simulink model "can8auto"  (R2018a)
settings: Solver=VariableStepAuto  StartTime=0.0  StopTime=5000  RelTol=1e-3
libraries: commcrc2 x20, simulink x20, simulink_extras x5, dspswit3 x5
(part 6 of 7)

== system can8auto/PDO NODO CAN /CAN NODE/NMT Frame generator/11-bit Adder/11-bit Adder/Full Adder5 ==
  A : Inport
  B : Inport  Port=2
  Cin : Inport  Port=3
  AND : Logic  IconShape=distinctive  AllPortsSameDT=off  OutDataTypeStr=boolean
  AND1 : Logic  IconShape=distinctive  AllPortsSameDT=off  OutDataTypeStr=boolean
  OR : Logic  Operator=OR  IconShape=distinctive  AllPortsSameDT=off  OutDataTypeStr=boolean
  XOR1 : Logic  Operator=XOR  IconShape=distinctive  AllPortsSameDT=off  OutDataTypeStr=boolean
  XOR2 : Logic  Operator=XOR  IconShape=distinctive  AllPortsSameDT=off  OutDataTypeStr=boolean
  S : Outport
  Cout : Outport  Port=2
  wires:
  AND/1 -> OR/1
  XOR2/1 -> S/1
  B/1 -> XOR1/2, AND1/2
  A/1 -> XOR1/1, AND1/1
  AND1/1 -> OR/2
  XOR1/1 -> XOR2/1, AND/2
  Cin/1 -> AND/1, XOR2/2
  OR/1 -> Cout/1

== system can8auto/PDO NODO CAN /CAN NODE/NMT Frame generator/11-bit Adder/11-bit Adder/Full Adder6 ==
  A : Inport
  B : Inport  Port=2
  Cin : Inport  Port=3
  AND : Logic  IconShape=distinctive  AllPortsSameDT=off  OutDataTypeStr=boolean
  AND1 : Logic  IconShape=distinctive  AllPortsSameDT=off  OutDataTypeStr=boolean
  OR : Logic  Operator=OR  IconShape=distinctive  AllPortsSameDT=off  OutDataTypeStr=boolean
  XOR1 : Logic  Operator=XOR  IconShape=distinctive  AllPortsSameDT=off  OutDataTypeStr=boolean
  XOR2 : Logic  Operator=XOR  IconShape=distinctive  AllPortsSameDT=off  OutDataTypeStr=boolean
  S : Outport
  Cout : Outport  Port=2
  wires:
  AND/1 -> OR/1
  XOR2/1 -> S/1
  B/1 -> XOR1/2, AND1/2
  A/1 -> XOR1/1, AND1/1
  AND1/1 -> OR/2
  XOR1/1 -> XOR2/1, AND/2
  Cin/1 -> AND/1, XOR2/2
  OR/1 -> Cout/1

== system can8auto/PDO NODO CAN /CAN NODE/NMT Frame generator/11-bit Adder/11-bit Adder/Full Adder7 ==
  A : Inport
  B : Inport  Port=2
  Cin : Inport  Port=3
  AND : Logic  IconShape=distinctive  AllPortsSameDT=off  OutDataTypeStr=boolean
  AND1 : Logic  IconShape=distinctive  AllPortsSameDT=off  OutDataTypeStr=boolean
  OR : Logic  Operator=OR  IconShape=distinctive  AllPortsSameDT=off  OutDataTypeStr=boolean
  XOR1 : Logic  Operator=XOR  IconShape=distinctive  AllPortsSameDT=off  OutDataTypeStr=boolean
  XOR2 : Logic  Operator=XOR  IconShape=distinctive  AllPortsSameDT=off  OutDataTypeStr=boolean
  S : Outport
  Cout : Outport  Port=2
  wires:
  AND/1 -> OR/1
  XOR2/1 -> S/1
  B/1 -> XOR1/2, AND1/2
  A/1 -> XOR1/1, AND1/1
  AND1/1 -> OR/2
  XOR1/1 -> XOR2/1, AND/2
  Cin/1 -> AND/1, XOR2/2
  OR/1 -> Cout/1

== system can8auto/PDO NODO CAN /CAN NODE/NMT Frame generator/11-bit Adder/11-bit Adder/Full Adder8 ==
  A : Inport
  B : Inport  Port=2
  Cin : Inport  Port=3
  AND : Logic  IconShape=distinctive  AllPortsSameDT=off  OutDataTypeStr=boolean
  AND1 : Logic  IconShape=distinctive  AllPortsSameDT=off  OutDataTypeStr=boolean
  OR : Logic  Operator=OR  IconShape=distinctive  AllPortsSameDT=off  OutDataTypeStr=boolean
  XOR1 : Logic  Operator=XOR  IconShape=distinctive  AllPortsSameDT=off  OutDataTypeStr=boolean
  XOR2 : Logic  Operator=XOR  IconShape=distinctive  AllPortsSameDT=off  OutDataTypeStr=boolean
  S : Outport
  Cout : Outport  Port=2
  wires:
  AND/1 -> OR/1
  XOR2/1 -> S/1
  B/1 -> XOR1/2, AND1/2
  A/1 -> XOR1/1, AND1/1
  AND1/1 -> OR/2
  XOR1/1 -> XOR2/1, AND/2
  Cin/1 -> AND/1, XOR2/2
  OR/1 -> Cout/1

== system can8auto/PDO NODO CAN /CAN NODE/NMT Frame generator/11-bit Adder/11-bit Adder/Full Adder9 ==
  A : Inport
  B : Inport  Port=2
  Cin : Inport  Port=3
  AND : Logic  IconShape=distinctive  AllPortsSameDT=off  OutDataTypeStr=boolean
  AND1 : Logic  IconShape=distinctive  AllPortsSameDT=off  OutDataTypeStr=boolean
  OR : Logic  Operator=OR  IconShape=distinctive  AllPortsSameDT=off  OutDataTypeStr=boolean
  XOR1 : Logic  Operator=XOR  IconShape=distinctive  AllPortsSameDT=off  OutDataTypeStr=boolean
  XOR2 : Logic  Operator=XOR  IconShape=distinctive  AllPortsSameDT=off  OutDataTypeStr=boolean
  S : Outport
  Cout : Outport  Port=2
  wires:
  AND/1 -> OR/1
  XOR2/1 -> S/1
  B/1 -> XOR1/2, AND1/2
  A/1 -> XOR1/1, AND1/1
  AND1/1 -> OR/2
  XOR1/1 -> XOR2/1, AND/2
  Cin/1 -> AND/1, XOR2/2
  OR/1 -> Cout/1

== system can8auto/PDO NODO CAN /CAN NODE/NMT Frame generator/11-bit Adder/11-bit Adder/Half Adder ==
  A : Inport
  B : Inport  Port=2
  AND : Logic  IconShape=distinctive  AllPortsSameDT=off  OutDataTypeStr=boolean
  XOR1 : Logic  Operator=XOR  IconShape=distinctive  AllPortsSameDT=off  OutDataTypeStr=boolean
  S : Outport
  C : Outport  Port=2
  wires:
  A/1 -> XOR1/1, AND/1
  B/1 -> XOR1/2, AND/2
  AND/1 -> C/1
  XOR1/1 -> S/1

== system can8auto/SDO NODO CAN/CAN NODE/Bootup Frame generator/11-bit Adder/8-bit Adder/Full Adder ==
  A : Inport
  B : Inport  Port=2
  Cin : Inport  Port=3
  AND : Logic  IconShape=distinctive  AllPortsSameDT=off  OutDataTypeStr=boolean
  AND1 : Logic  IconShape=distinctive  AllPortsSameDT=off  OutDataTypeStr=boolean
  OR : Logic  Operator=OR  IconShape=distinctive  AllPortsSameDT=off  OutDataTypeStr=boolean
  XOR1 : Logic  Operator=XOR  IconShape=distinctive  AllPortsSameDT=off  OutDataTypeStr=boolean
  XOR2 : Logic  Operator=XOR  IconShape=distinctive  AllPortsSameDT=off  OutDataTypeStr=boolean
  S : Outport
  Cout : Outport  Port=2
  wires:
  AND/1 -> OR/1
  XOR2/1 -> S/1
  B/1 -> XOR1/2, AND1/2
  A/1 -> XOR1/1, AND1/1
  AND1/1 -> OR/2
  XOR1/1 -> XOR2/1, AND/2
  Cin/1 -> AND/1, XOR2/2
  OR/1 -> Cout/1

== system can8auto/SDO NODO CAN/CAN NODE/Bootup Frame generator/11-bit Adder/8-bit Adder/Full Adder1 ==
  A : Inport
  B : Inport  Port=2
  Cin : Inport  Port=3
  AND : Logic  IconShape=distinctive  AllPortsSameDT=off  OutDataTypeStr=boolean
  AND1 : Logic  IconShape=distinctive  AllPortsSameDT=off  OutDataTypeStr=boolean
  OR : Logic  Operator=OR  IconShape=distinctive  AllPortsSameDT=off  OutDataTypeStr=boolean
  XOR1 : Logic  Operator=XOR  IconShape=distinctive  AllPortsSameDT=off  OutDataTypeStr=boolean
  XOR2 : Logic  Operator=XOR  IconShape=distinctive  AllPortsSameDT=off  OutDataTypeStr=boolean
  S : Outport
  Cout : Outport  Port=2
  wires:
  AND/1 -> OR/1
  XOR2/1 -> S/1
  B/1 -> XOR1/2, AND1/2
  A/1 -> XOR1/1, AND1/1
  AND1/1 -> OR/2
  XOR1/1 -> XOR2/1, AND/2
  Cin/1 -> AND/1, XOR2/2
  OR/1 -> Cout/1

== system can8auto/SDO NODO CAN/CAN NODE/Bootup Frame generator/11-bit Adder/8-bit Adder/Full Adder2 ==
  A : Inport
  B : Inport  Port=2
  Cin : Inport  Port=3
  AND : Logic  IconShape=distinctive  AllPortsSameDT=off  OutDataTypeStr=boolean
  AND1 : Logic  IconShape=distinctive  AllPortsSameDT=off  OutDataTypeStr=boolean
  OR : Logic  Operator=OR  IconShape=distinctive  AllPortsSameDT=off  OutDataTypeStr=boolean
  XOR1 : Logic  Operator=XOR  IconShape=distinctive  AllPortsSameDT=off  OutDataTypeStr=boolean
  XOR2 : Logic  Operator=XOR  IconShape=distinctive  AllPortsSameDT=off  OutDataTypeStr=boolean
  S : Outport
  Cout : Outport  Port=2
  wires:
  AND/1 -> OR/1
  XOR2/1 -> S/1
  B/1 -> XOR1/2, AND1/2
  A/1 -> XOR1/1, AND1/1
  AND1/1 -> OR/2
  XOR1/1 -> XOR2/1, AND/2
  Cin/1 -> AND/1, XOR2/2
  OR/1 -> Cout/1

== system can8auto/SDO NODO CAN/CAN NODE/Bootup Frame generator/11-bit Adder/8-bit Adder/Full Adder3 ==
  A : Inport
  B : Inport  Port=2
  Cin : Inport  Port=3
  AND : Logic  IconShape=distinctive  AllPortsSameDT=off  OutDataTypeStr=boolean
  AND1 : Logic  IconShape=distinctive  AllPortsSameDT=off  OutDataTypeStr=boolean
  OR : Logic  Operator=OR  IconShape=distinctive  AllPortsSameDT=off  OutDataTypeStr=boolean
  XOR1 : Logic  Operator=XOR  IconShape=distinctive  AllPortsSameDT=off  OutDataTypeStr=boolean
  XOR2 : Logic  Operator=XOR  IconShape=distinctive  AllPortsSameDT=off  OutDataTypeStr=boolean
  S : Outport
  Cout : Outport  Port=2
  wires:
  AND/1 -> OR/1
  XOR2/1 -> S/1
  B/1 -> XOR1/2, AND1/2
  A/1 -> XOR1/1, AND1/1
  AND1/1 -> OR/2
  XOR1/1 -> XOR2/1, AND/2
  Cin/1 -> AND/1, XOR2/2
  OR/1 -> Cout/1

== system can8auto/SDO NODO CAN/CAN NODE/Bootup Frame generator/11-bit Adder/8-bit Adder/Full Adder4 ==
  A : Inport
  B : Inport  Port=2
  Cin : Inport  Port=3
  AND : Logic  IconShape=distinctive  AllPortsSameDT=off  OutDataTypeStr=boolean
  AND1 : Logic  IconShape=distinctive  AllPortsSameDT=off  OutDataTypeStr=boolean
  OR : Logic  Operator=OR  IconShape=distinctive  AllPortsSameDT=off  OutDataTypeStr=boolean
  XOR1 : Logic  Operator=XOR  IconShape=distinctive  AllPortsSameDT=off  OutDataTypeStr=boolean
  XOR2 : Logic  Operator=XOR  IconShape=distinctive  AllPortsSameDT=off  OutDataTypeStr=boolean
  S : Outport
  Cout : Outport  Port=2
  wires:
  AND/1 -> OR/1
  XOR2/1 -> S/1
  B/1 -> XOR1/2, AND1/2
  A/1 -> XOR1/1, AND1/1
  AND1/1 -> OR/2
  XOR1/1 -> XOR2/1, AND/2
  Cin/1 -> AND/1, XOR2/2
  OR/1 -> Cout/1

== system can8auto/SDO NODO CAN/CAN NODE/Bootup Frame generator/11-bit Adder/8-bit Adder/Full Adder5 ==
  A : Inport
  B : Inport  Port=2
  Cin : Inport  Port=3
  AND : Logic  IconShape=distinctive  AllPortsSameDT=off  OutDataTypeStr=boolean
  AND1 : Logic  IconShape=distinctive  AllPortsSameDT=off  OutDataTypeStr=boolean
  OR : Logic  Operator=OR  IconShape=distinctive  AllPortsSameDT=off  OutDataTypeStr=boolean
  XOR1 : Logic  Operator=XOR  IconShape=distinctive  AllPortsSameDT=off  OutDataTypeStr=boolean
  XOR2 : Logic  Operator=XOR  IconShape=distinctive  AllPortsSameDT=off  OutDataTypeStr=boolean
  S : Outport
  Cout : Outport  Port=2
  wires:
  AND/1 -> OR/1
  XOR2/1 -> S/1
  B/1 -> XOR1/2, AND1/2
  A/1 -> XOR1/1, AND1/1
  AND1/1 -> OR/2
  XOR1/1 -> XOR2/1, AND/2
  Cin/1 -> AND/1, XOR2/2
  OR/1 -> Cout/1

== system can8auto/SDO NODO CAN/CAN NODE/Bootup Frame generator/11-bit Adder/8-bit Adder/Full Adder6 ==
  A : Inport
  B : Inport  Port=2
  Cin : Inport  Port=3
  AND : Logic  IconShape=distinctive  AllPortsSameDT=off  OutDataTypeStr=boolean
  AND1 : Logic  IconShape=distinctive  AllPortsSameDT=off  OutDataTypeStr=boolean
  OR : Logic  Operator=OR  IconShape=distinctive  AllPortsSameDT=off  OutDataTypeStr=boolean
  XOR1 : Logic  Operator=XOR  IconShape=distinctive  AllPortsSameDT=off  OutDataTypeStr=boolean
  XOR2 : Logic  Operator=XOR  IconShape=distinctive  AllPortsSameDT=off  OutDataTypeStr=boolean
  S : Outport
  Cout : Outport  Port=2
  wires:
  AND/1 -> OR/1
  XOR2/1 -> S/1
  B/1 -> XOR1/2, AND1/2
  A/1 -> XOR1/1, AND1/1
  AND1/1 -> OR/2
  XOR1/1 -> XOR2/1, AND/2
  Cin/1 -> AND/1, XOR2/2
  OR/1 -> Cout/1

== system can8auto/SDO NODO CAN/CAN NODE/Bootup Frame generator/11-bit Adder/8-bit Adder/Full Adder7 ==
  A : Inport
  B : Inport  Port=2
  Cin : Inport  Port=3
  AND : Logic  IconShape=distinctive  AllPortsSameDT=off  OutDataTypeStr=boolean
  AND1 : Logic  IconShape=distinctive  AllPortsSameDT=off  OutDataTypeStr=boolean
  OR : Logic  Operator=OR  IconShape=distinctive  AllPortsSameDT=off  OutDataTypeStr=boolean
  XOR1 : Logic  Operator=XOR  IconShape=distinctive  AllPortsSameDT=off  OutDataTypeStr=boolean
  XOR2 : Logic  Operator=XOR  IconShape=distinctive  AllPortsSameDT=off  OutDataTypeStr=boolean
  S : Outport
  Cout : Outport  Port=2
  wires:
  AND/1 -> OR/1
  XOR2/1 -> S/1
  B/1 -> XOR1/2, AND1/2
  A/1 -> XOR1/1, AND1/1
  AND1/1 -> OR/2
  XOR1/1 -> XOR2/1, AND/2
  Cin/1 -> AND/1, XOR2/2
  OR/1 -> Cout/1

== system can8auto/SDO NODO CAN/CAN NODE/Bootup Frame generator/11-bit Adder/8-bit Adder/Full Adder8 ==
  A : Inport
  B : Inport  Port=2
  Cin : Inport  Port=3
  AND : Logic  IconShape=distinctive  AllPortsSameDT=off  OutDataTypeStr=boolean
  AND1 : Logic  IconShape=distinctive  AllPortsSameDT=off  OutDataTypeStr=boolean
  OR : Logic  Operator=OR  IconShape=distinctive  AllPortsSameDT=off  OutDataTypeStr=boolean
  XOR1 : Logic  Operator=XOR  IconShape=distinctive  AllPortsSameDT=off  OutDataTypeStr=boolean
  XOR2 : Logic  Operator=XOR  IconShape=distinctive  AllPortsSameDT=off  OutDataTypeStr=boolean
  S : Outport
  Cout : Outport  Port=2
  wires:
  AND/1 -> OR/1
  XOR2/1 -> S/1
  B/1 -> XOR1/2, AND1/2
  A/1 -> XOR1/1, AND1/1
  AND1/1 -> OR/2
  XOR1/1 -> XOR2/1, AND/2
  Cin/1 -> AND/1, XOR2/2
  OR/1 -> Cout/1

== system can8auto/SDO NODO CAN/CAN NODE/Bootup Frame generator/11-bit Adder/8-bit Adder/Full Adder9 ==
  A : Inport
  B : Inport  Port=2
  Cin : Inport  Port=3
  AND : Logic  IconShape=distinctive  AllPortsSameDT=off  OutDataTypeStr=boolean
  AND1 : Logic  IconShape=distinctive  AllPortsSameDT=off  OutDataTypeStr=boolean
  OR : Logic  Operator=OR  IconShape=distinctive  AllPortsSameDT=off  OutDataTypeStr=boolean
  XOR1 : Logic  Operator=XOR  IconShape=distinctive  AllPortsSameDT=off  OutDataTypeStr=boolean
  XOR2 : Logic  Operator=XOR  IconShape=distinctive  AllPortsSameDT=off  OutDataTypeStr=boolean
  S : Outport
  Cout : Outport  Port=2
  wires:
  AND/1 -> OR/1
  XOR2/1 -> S/1
  B/1 -> XOR1/2, AND1/2
  A/1 -> XOR1/1, AND1/1
  AND1/1 -> OR/2
  XOR1/1 -> XOR2/1, AND/2
  Cin/1 -> AND/1, XOR2/2
  OR/1 -> Cout/1

== system can8auto/SDO NODO CAN/CAN NODE/Bootup Frame generator/11-bit Adder/8-bit Adder/Half Adder ==
  A : Inport
  B : Inport  Port=2
  AND : Logic  IconShape=distinctive  AllPortsSameDT=off  OutDataTypeStr=boolean
  XOR1 : Logic  Operator=XOR  IconShape=distinctive  AllPortsSameDT=off  OutDataTypeStr=boolean
  S : Outport
  C : Outport  Port=2
  wires:
  A/1 -> XOR1/1, AND/1
  B/1 -> XOR1/2, AND/2
  AND/1 -> C/1
  XOR1/1 -> S/1

== system can8auto/SDO NODO CAN/CAN NODE/NMT Frame generator/11-bit Adder/11-bit Adder/Full Adder ==
  A : Inport
  B : Inport  Port=2
  Cin : Inport  Port=3
  AND : Logic  IconShape=distinctive  AllPortsSameDT=off  OutDataTypeStr=boolean
  AND1 : Logic  IconShape=distinctive  AllPortsSameDT=off  OutDataTypeStr=boolean
  OR : Logic  Operator=OR  IconShape=distinctive  AllPortsSameDT=off  OutDataTypeStr=boolean
  XOR1 : Logic  Operator=XOR  IconShape=distinctive  AllPortsSameDT=off  OutDataTypeStr=boolean
  XOR2 : Logic  Operator=XOR  IconShape=distinctive  AllPortsSameDT=off  OutDataTypeStr=boolean
  S : Outport
  Cout : Outport  Port=2
  wires:
  AND/1 -> OR/1
  XOR2/1 -> S/1
  B/1 -> XOR1/2, AND1/2
  A/1 -> XOR1/1, AND1/1
  AND1/1 -> OR/2
  XOR1/1 -> XOR2/1, AND/2
  Cin/1 -> AND/1, XOR2/2
  OR/1 -> Cout/1

== system can8auto/SDO NODO CAN/CAN NODE/NMT Frame generator/11-bit Adder/11-bit Adder/Full Adder1 ==
  A : Inport
  B : Inport  Port=2
  Cin : Inport  Port=3
  AND : Logic  IconShape=distinctive  AllPortsSameDT=off  OutDataTypeStr=boolean
  AND1 : Logic  IconShape=distinctive  AllPortsSameDT=off  OutDataTypeStr=boolean
  OR : Logic  Operator=OR  IconShape=distinctive  AllPortsSameDT=off  OutDataTypeStr=boolean
  XOR1 : Logic  Operator=XOR  IconShape=distinctive  AllPortsSameDT=off  OutDataTypeStr=boolean
  XOR2 : Logic  Operator=XOR  IconShape=distinctive  AllPortsSameDT=off  OutDataTypeStr=boolean
  S : Outport
  Cout : Outport  Port=2
  wires:
  AND/1 -> OR/1
  XOR2/1 -> S/1
  B/1 -> XOR1/2, AND1/2
  A/1 -> XOR1/1, AND1/1
  AND1/1 -> OR/2
  XOR1/1 -> XOR2/1, AND/2
  Cin/1 -> AND/1, XOR2/2
  OR/1 -> Cout/1

== system can8auto/SDO NODO CAN/CAN NODE/NMT Frame generator/11-bit Adder/11-bit Adder/Full Adder2 ==
  A : Inport
  B : Inport  Port=2
  Cin : Inport  Port=3
  AND : Logic  IconShape=distinctive  AllPortsSameDT=off  OutDataTypeStr=boolean
  AND1 : Logic  IconShape=distinctive  AllPortsSameDT=off  OutDataTypeStr=boolean
  OR : Logic  Operator=OR  IconShape=distinctive  AllPortsSameDT=off  OutDataTypeStr=boolean
  XOR1 : Logic  Operator=XOR  IconShape=distinctive  AllPortsSameDT=off  OutDataTypeStr=boolean
  XOR2 : Logic  Operator=XOR  IconShape=distinctive  AllPortsSameDT=off  OutDataTypeStr=boolean
  S : Outport
  Cout : Outport  Port=2
  wires:
  AND/1 -> OR/1
  XOR2/1 -> S/1
  B/1 -> XOR1/2, AND1/2
  A/1 -> XOR1/1, AND1/1
  AND1/1 -> OR/2
  XOR1/1 -> XOR2/1, AND/2
  Cin/1 -> AND/1, XOR2/2
  OR/1 -> Cout/1

== system can8auto/SDO NODO CAN/CAN NODE/NMT Frame generator/11-bit Adder/11-bit Adder/Full Adder3 ==
  A : Inport
  B : Inport  Port=2
  Cin : Inport  Port=3
  AND : Logic  IconShape=distinctive  AllPortsSameDT=off  OutDataTypeStr=boolean
  AND1 : Logic  IconShape=distinctive  AllPortsSameDT=off  OutDataTypeStr=boolean
  OR : Logic  Operator=OR  IconShape=distinctive  AllPortsSameDT=off  OutDataTypeStr=boolean
  XOR1 : Logic  Operator=XOR  IconShape=distinctive  AllPortsSameDT=off  OutDataTypeStr=boolean
  XOR2 : Logic  Operator=XOR  IconShape=distinctive  AllPortsSameDT=off  OutDataTypeStr=boolean
  S : Outport
  Cout : Outport  Port=2
  wires:
  AND/1 -> OR/1
  XOR2/1 -> S/1
  B/1 -> XOR1/2, AND1/2
  A/1 -> XOR1/1, AND1/1
  AND1/1 -> OR/2
  XOR1/1 -> XOR2/1, AND/2
  Cin/1 -> AND/1, XOR2/2
  OR/1 -> Cout/1

== system can8auto/SDO NODO CAN/CAN NODE/NMT Frame generator/11-bit Adder/11-bit Adder/Full Adder4 ==
  A : Inport
  B : Inport  Port=2
  Cin : Inport  Port=3
  AND : Logic  IconShape=distinctive  AllPortsSameDT=off  OutDataTypeStr=boolean
  AND1 : Logic  IconShape=distinctive  AllPortsSameDT=off  OutDataTypeStr=boolean
  OR : Logic  Operator=OR  IconShape=distinctive  AllPortsSameDT=off  OutDataTypeStr=boolean
  XOR1 : Logic  Operator=XOR  IconShape=distinctive  AllPortsSameDT=off  OutDataTypeStr=boolean
  XOR2 : Logic  Operator=XOR  IconShape=distinctive  AllPortsSameDT=off  OutDataTypeStr=boolean
  S : Outport
  Cout : Outport  Port=2
  wires:
  AND/1 -> OR/1
  XOR2/1 -> S/1
  B/1 -> XOR1/2, AND1/2
  A/1 -> XOR1/1, AND1/1
  AND1/1 -> OR/2
  XOR1/1 -> XOR2/1, AND/2
  Cin/1 -> AND/1, XOR2/2
  OR/1 -> Cout/1

== system can8auto/SDO NODO CAN/CAN NODE/NMT Frame generator/11-bit Adder/11-bit Adder/Full Adder5 ==
  A : Inport
  B : Inport  Port=2
  Cin : Inport  Port=3
  AND : Logic  IconShape=distinctive  AllPortsSameDT=off  OutDataTypeStr=boolean
  AND1 : Logic  IconShape=distinctive  AllPortsSameDT=off  OutDataTypeStr=boolean
  OR : Logic  Operator=OR  IconShape=distinctive  AllPortsSameDT=off  OutDataTypeStr=boolean
  XOR1 : Logic  Operator=XOR  IconShape=distinctive  AllPortsSameDT=off  OutDataTypeStr=boolean
  XOR2 : Logic  Operator=XOR  IconShape=distinctive  AllPortsSameDT=off  OutDataTypeStr=boolean
  S : Outport
  Cout : Outport  Port=2
  wires:
  AND/1 -> OR/1
  XOR2/1 -> S/1
  B/1 -> XOR1/2, AND1/2
  A/1 -> XOR1/1, AND1/1
  AND1/1 -> OR/2
  XOR1/1 -> XOR2/1, AND/2
  Cin/1 -> AND/1, XOR2/2
  OR/1 -> Cout/1

== system can8auto/SDO NODO CAN/CAN NODE/NMT Frame generator/11-bit Adder/11-bit Adder/Full Adder6 ==
  A : Inport
  B : Inport  Port=2
  Cin : Inport  Port=3
  AND : Logic  IconShape=distinctive  AllPortsSameDT=off  OutDataTypeStr=boolean
  AND1 : Logic  IconShape=distinctive  AllPortsSameDT=off  OutDataTypeStr=boolean
  OR : Logic  Operator=OR  IconShape=distinctive  AllPortsSameDT=off  OutDataTypeStr=boolean
  XOR1 : Logic  Operator=XOR  IconShape=distinctive  AllPortsSameDT=off  OutDataTypeStr=boolean
  XOR2 : Logic  Operator=XOR  IconShape=distinctive  AllPortsSameDT=off  OutDataTypeStr=boolean
  S : Outport
  Cout : Outport  Port=2
  wires:
  AND/1 -> OR/1
  XOR2/1 -> S/1
  B/1 -> XOR1/2, AND1/2
  A/1 -> XOR1/1, AND1/1
  AND1/1 -> OR/2
  XOR1/1 -> XOR2/1, AND/2
  Cin/1 -> AND/1, XOR2/2
  OR/1 -> Cout/1

== system can8auto/SDO NODO CAN/CAN NODE/NMT Frame generator/11-bit Adder/11-bit Adder/Full Adder7 ==
  A : Inport
  B : Inport  Port=2
  Cin : Inport  Port=3
  AND : Logic  IconShape=distinctive  AllPortsSameDT=off  OutDataTypeStr=boolean
  AND1 : Logic  IconShape=distinctive  AllPortsSameDT=off  OutDataTypeStr=boolean
  OR : Logic  Operator=OR  IconShape=distinctive  AllPortsSameDT=off  OutDataTypeStr=boolean
  XOR1 : Logic  Operator=XOR  IconShape=distinctive  AllPortsSameDT=off  OutDataTypeStr=boolean
  XOR2 : Logic  Operator=XOR  IconShape=distinctive  AllPortsSameDT=off  OutDataTypeStr=boolean
  S : Outport
  Cout : Outport  Port=2
  wires:
  AND/1 -> OR/1
  XOR2/1 -> S/1
  B/1 -> XOR1/2, AND1/2
  A/1 -> XOR1/1, AND1/1
  AND1/1 -> OR/2
  XOR1/1 -> XOR2/1, AND/2
  Cin/1 -> AND/1, XOR2/2
  OR/1 -> Cout/1

== system can8auto/SDO NODO CAN/CAN NODE/NMT Frame generator/11-bit Adder/11-bit Adder/Full Adder8 ==
  A : Inport
  B : Inport  Port=2
  Cin : Inport  Port=3
  AND : Logic  IconShape=distinctive  AllPortsSameDT=off  OutDataTypeStr=boolean
  AND1 : Logic  IconShape=distinctive  AllPortsSameDT=off  OutDataTypeStr=boolean
  OR : Logic  Operator=OR  IconShape=distinctive  AllPortsSameDT=off  OutDataTypeStr=boolean
  XOR1 : Logic  Operator=XOR  IconShape=distinctive  AllPortsSameDT=off  OutDataTypeStr=boolean
  XOR2 : Logic  Operator=XOR  IconShape=distinctive  AllPortsSameDT=off  OutDataTypeStr=boolean
  S : Outport
  Cout : Outport  Port=2
  wires:
  AND/1 -> OR/1
  XOR2/1 -> S/1
  B/1 -> XOR1/2, AND1/2
  A/1 -> XOR1/1, AND1/1
  AND1/1 -> OR/2
  XOR1/1 -> XOR2/1, AND/2
  Cin/1 -> AND/1, XOR2/2
  OR/1 -> Cout/1

== system can8auto/SDO NODO CAN/CAN NODE/NMT Frame generator/11-bit Adder/11-bit Adder/Full Adder9 ==
  A : Inport
  B : Inport  Port=2
  Cin : Inport  Port=3
  AND : Logic  IconShape=distinctive  AllPortsSameDT=off  OutDataTypeStr=boolean
  AND1 : Logic  IconShape=distinctive  AllPortsSameDT=off  OutDataTypeStr=boolean
  OR : Logic  Operator=OR  IconShape=distinctive  AllPortsSameDT=off  OutDataTypeStr=boolean
  XOR1 : Logic  Operator=XOR  IconShape=distinctive  AllPortsSameDT=off  OutDataTypeStr=boolean
  XOR2 : Logic  Operator=XOR  IconShape=distinctive  AllPortsSameDT=off  OutDataTypeStr=boolean
  S : Outport
  Cout : Outport  Port=2
  wires:
  AND/1 -> OR/1
  XOR2/1 -> S/1
  B/1 -> XOR1/2, AND1/2
  A/1 -> XOR1/1, AND1/1
  AND1/1 -> OR/2
  XOR1/1 -> XOR2/1, AND/2
  Cin/1 -> AND/1, XOR2/2
  OR/1 -> Cout/1

== system can8auto/SDO NODO CAN/CAN NODE/NMT Frame generator/11-bit Adder/11-bit Adder/Half Adder ==
  A : Inport
  B : Inport  Port=2
  AND : Logic  IconShape=distinctive  AllPortsSameDT=off  OutDataTypeStr=boolean
  XOR1 : Logic  Operator=XOR  IconShape=distinctive  AllPortsSameDT=off  OutDataTypeStr=boolean
  S : Outport
  C : Outport  Port=2
  wires:
  A/1 -> XOR1/1, AND/1
  B/1 -> XOR1/2, AND/2
  AND/1 -> C/1
  XOR1/1 -> S/1

== system can8auto/SYNC PRODUCER/CAN NODE/Bootup Frame generator/11-bit Adder/8-bit Adder/Full Adder ==
  A : Inport
  B : Inport  Port=2
  Cin : Inport  Port=3
  AND : Logic  IconShape=distinctive  AllPortsSameDT=off  OutDataTypeStr=boolean
  AND1 : Logic  IconShape=distinctive  AllPortsSameDT=off  OutDataTypeStr=boolean
  OR : Logic  Operator=OR  IconShape=distinctive  AllPortsSameDT=off  OutDataTypeStr=boolean
  XOR1 : Logic  Operator=XOR  IconShape=distinctive  AllPortsSameDT=off  OutDataTypeStr=boolean
  XOR2 : Logic  Operator=XOR  IconShape=distinctive  AllPortsSameDT=off  OutDataTypeStr=boolean
  S : Outport
  Cout : Outport  Port=2
  wires:
  AND/1 -> OR/1
  XOR2/1 -> S/1
  B/1 -> XOR1/2, AND1/2
  A/1 -> XOR1/1, AND1/1
  AND1/1 -> OR/2
  XOR1/1 -> XOR2/1, AND/2
  Cin/1 -> AND/1, XOR2/2
  OR/1 -> Cout/1

== system can8auto/SYNC PRODUCER/CAN NODE/Bootup Frame generator/11-bit Adder/8-bit Adder/Full Adder1 ==
  A : Inport
  B : Inport  Port=2
  Cin : Inport  Port=3
  AND : Logic  IconShape=distinctive  AllPortsSameDT=off  OutDataTypeStr=boolean
  AND1 : Logic  IconShape=distinctive  AllPortsSameDT=off  OutDataTypeStr=boolean
  OR : Logic  Operator=OR  IconShape=distinctive  AllPortsSameDT=off  OutDataTypeStr=boolean
  XOR1 : Logic  Operator=XOR  IconShape=distinctive  AllPortsSameDT=off  OutDataTypeStr=boolean
  XOR2 : Logic  Operator=XOR  IconShape=distinctive  AllPortsSameDT=off  OutDataTypeStr=boolean
  S : Outport
  Cout : Outport  Port=2
  wires:
  AND/1 -> OR/1
  XOR2/1 -> S/1
  B/1 -> XOR1/2, AND1/2
  A/1 -> XOR1/1, AND1/1
  AND1/1 -> OR/2
  XOR1/1 -> XOR2/1, AND/2
  Cin/1 -> AND/1, XOR2/2
  OR/1 -> Cout/1

== system can8auto/SYNC PRODUCER/CAN NODE/Bootup Frame generator/11-bit Adder/8-bit Adder/Full Adder2 ==
  A : Inport
  B : Inport  Port=2
  Cin : Inport  Port=3
  AND : Logic  IconShape=distinctive  AllPortsSameDT=off  OutDataTypeStr=boolean
  AND1 : Logic  IconShape=distinctive  AllPortsSameDT=off  OutDataTypeStr=boolean
  OR : Logic  Operator=OR  IconShape=distinctive  AllPortsSameDT=off  OutDataTypeStr=boolean
  XOR1 : Logic  Operator=XOR  IconShape=distinctive  AllPortsSameDT=off  OutDataTypeStr=boolean
  XOR2 : Logic  Operator=XOR  IconShape=distinctive  AllPortsSameDT=off  OutDataTypeStr=boolean
  S : Outport
  Cout : Outport  Port=2
  wires:
  AND/1 -> OR/1
  XOR2/1 -> S/1
  B/1 -> XOR1/2, AND1/2
  A/1 -> XOR1/1, AND1/1
  AND1/1 -> OR/2
  XOR1/1 -> XOR2/1, AND/2
  Cin/1 -> AND/1, XOR2/2
  OR/1 -> Cout/1

== system can8auto/SYNC PRODUCER/CAN NODE/Bootup Frame generator/11-bit Adder/8-bit Adder/Full Adder3 ==
  A : Inport
  B : Inport  Port=2
  Cin : Inport  Port=3
  AND : Logic  IconShape=distinctive  AllPortsSameDT=off  OutDataTypeStr=boolean
  AND1 : Logic  IconShape=distinctive  AllPortsSameDT=off  OutDataTypeStr=boolean
  OR : Logic  Operator=OR  IconShape=distinctive  AllPortsSameDT=off  OutDataTypeStr=boolean
  XOR1 : Logic  Operator=XOR  IconShape=distinctive  AllPortsSameDT=off  OutDataTypeStr=boolean
  XOR2 : Logic  Operator=XOR  IconShape=distinctive  AllPortsSameDT=off  OutDataTypeStr=boolean
  S : Outport
  Cout : Outport  Port=2
  wires:
  AND/1 -> OR/1
  XOR2/1 -> S/1
  B/1 -> XOR1/2, AND1/2
  A/1 -> XOR1/1, AND1/1
  AND1/1 -> OR/2
  XOR1/1 -> XOR2/1, AND/2
  Cin/1 -> AND/1, XOR2/2
  OR/1 -> Cout/1

== system can8auto/SYNC PRODUCER/CAN NODE/Bootup Frame generator/11-bit Adder/8-bit Adder/Full Adder4 ==
  A : Inport
  B : Inport  Port=2
  Cin : Inport  Port=3
  AND : Logic  IconShape=distinctive  AllPortsSameDT=off  OutDataTypeStr=boolean
  AND1 : Logic  IconShape=distinctive  AllPortsSameDT=off  OutDataTypeStr=boolean
  OR : Logic  Operator=OR  IconShape=distinctive  AllPortsSameDT=off  OutDataTypeStr=boolean
  XOR1 : Logic  Operator=XOR  IconShape=distinctive  AllPortsSameDT=off  OutDataTypeStr=boolean
  XOR2 : Logic  Operator=XOR  IconShape=distinctive  AllPortsSameDT=off  OutDataTypeStr=boolean
  S : Outport
  Cout : Outport  Port=2
  wires:
  AND/1 -> OR/1
  XOR2/1 -> S/1
  B/1 -> XOR1/2, AND1/2
  A/1 -> XOR1/1, AND1/1
  AND1/1 -> OR/2
  XOR1/1 -> XOR2/1, AND/2
  Cin/1 -> AND/1, XOR2/2
  OR/1 -> Cout/1

== system can8auto/SYNC PRODUCER/CAN NODE/Bootup Frame generator/11-bit Adder/8-bit Adder/Full Adder5 ==
  A : Inport
  B : Inport  Port=2
  Cin : Inport  Port=3
  AND : Logic  IconShape=distinctive  AllPortsSameDT=off  OutDataTypeStr=boolean
  AND1 : Logic  IconShape=distinctive  AllPortsSameDT=off  OutDataTypeStr=boolean
  OR : Logic  Operator=OR  IconShape=distinctive  AllPortsSameDT=off  OutDataTypeStr=boolean
  XOR1 : Logic  Operator=XOR  IconShape=distinctive  AllPortsSameDT=off  OutDataTypeStr=boolean
  XOR2 : Logic  Operator=XOR  IconShape=distinctive  AllPortsSameDT=off  OutDataTypeStr=boolean
  S : Outport
  Cout : Outport  Port=2
  wires:
  AND/1 -> OR/1
  XOR2/1 -> S/1
  B/1 -> XOR1/2, AND1/2
  A/1 -> XOR1/1, AND1/1
  AND1/1 -> OR/2
  XOR1/1 -> XOR2/1, AND/2
  Cin/1 -> AND/1, XOR2/2
  OR/1 -> Cout/1

== system can8auto/SYNC PRODUCER/CAN NODE/Bootup Frame generator/11-bit Adder/8-bit Adder/Full Adder6 ==
  A : Inport
  B : Inport  Port=2
  Cin : Inport  Port=3
  AND : Logic  IconShape=distinctive  AllPortsSameDT=off  OutDataTypeStr=boolean
  AND1 : Logic  IconShape=distinctive  AllPortsSameDT=off  OutDataTypeStr=boolean
  OR : Logic  Operator=OR  IconShape=distinctive  AllPortsSameDT=off  OutDataTypeStr=boolean
  XOR1 : Logic  Operator=XOR  IconShape=distinctive  AllPortsSameDT=off  OutDataTypeStr=boolean
  XOR2 : Logic  Operator=XOR  IconShape=distinctive  AllPortsSameDT=off  OutDataTypeStr=boolean
  S : Outport
  Cout : Outport  Port=2
  wires:
  AND/1 -> OR/1
  XOR2/1 -> S/1
  B/1 -> XOR1/2, AND1/2
  A/1 -> XOR1/1, AND1/1
  AND1/1 -> OR/2
  XOR1/1 -> XOR2/1, AND/2
  Cin/1 -> AND/1, XOR2/2
  OR/1 -> Cout/1

== system can8auto/SYNC PRODUCER/CAN NODE/Bootup Frame generator/11-bit Adder/8-bit Adder/Full Adder7 ==
  A : Inport
  B : Inport  Port=2
  Cin : Inport  Port=3
  AND : Logic  IconShape=distinctive  AllPortsSameDT=off  OutDataTypeStr=boolean
  AND1 : Logic  IconShape=distinctive  AllPortsSameDT=off  OutDataTypeStr=boolean
  OR : Logic  Operator=OR  IconShape=distinctive  AllPortsSameDT=off  OutDataTypeStr=boolean
  XOR1 : Logic  Operator=XOR  IconShape=distinctive  AllPortsSameDT=off  OutDataTypeStr=boolean
  XOR2 : Logic  Operator=XOR  IconShape=distinctive  AllPortsSameDT=off  OutDataTypeStr=boolean
  S : Outport
  Cout : Outport  Port=2
  wires:
  AND/1 -> OR/1
  XOR2/1 -> S/1
  B/1 -> XOR1/2, AND1/2
  A/1 -> XOR1/1, AND1/1
  AND1/1 -> OR/2
  XOR1/1 -> XOR2/1, AND/2
  Cin/1 -> AND/1, XOR2/2
  OR/1 -> Cout/1

== system can8auto/SYNC PRODUCER/CAN NODE/Bootup Frame generator/11-bit Adder/8-bit Adder/Full Adder8 ==
  A : Inport
  B : Inport  Port=2
  Cin : Inport  Port=3
  AND : Logic  IconShape=distinctive  AllPortsSameDT=off  OutDataTypeStr=boolean
  AND1 : Logic  IconShape=distinctive  AllPortsSameDT=off  OutDataTypeStr=boolean
  OR : Logic  Operator=OR  IconShape=distinctive  AllPortsSameDT=off  OutDataTypeStr=boolean
  XOR1 : Logic  Operator=XOR  IconShape=distinctive  AllPortsSameDT=off  OutDataTypeStr=boolean
  XOR2 : Logic  Operator=XOR  IconShape=distinctive  AllPortsSameDT=off  OutDataTypeStr=boolean
  S : Outport
  Cout : Outport  Port=2
  wires:
  AND/1 -> OR/1
  XOR2/1 -> S/1
  B/1 -> XOR1/2, AND1/2
  A/1 -> XOR1/1, AND1/1
  AND1/1 -> OR/2
  XOR1/1 -> XOR2/1, AND/2
  Cin/1 -> AND/1, XOR2/2
  OR/1 -> Cout/1

== system can8auto/SYNC PRODUCER/CAN NODE/Bootup Frame generator/11-bit Adder/8-bit Adder/Full Adder9 ==
  A : Inport
  B : Inport  Port=2
  Cin : Inport  Port=3
  AND : Logic  IconShape=distinctive  AllPortsSameDT=off  OutDataTypeStr=boolean
  AND1 : Logic  IconShape=distinctive  AllPortsSameDT=off  OutDataTypeStr=boolean
  OR : Logic  Operator=OR  IconShape=distinctive  AllPortsSameDT=off  OutDataTypeStr=boolean
  XOR1 : Logic  Operator=XOR  IconShape=distinctive  AllPortsSameDT=off  OutDataTypeStr=boolean
  XOR2 : Logic  Operator=XOR  IconShape=distinctive  AllPortsSameDT=off  OutDataTypeStr=boolean
  S : Outport
  Cout : Outport  Port=2
  wires:
  AND/1 -> OR/1
  XOR2/1 -> S/1
  B/1 -> XOR1/2, AND1/2
  A/1 -> XOR1/1, AND1/1
  AND1/1 -> OR/2
  XOR1/1 -> XOR2/1, AND/2
  Cin/1 -> AND/1, XOR2/2
  OR/1 -> Cout/1

== system can8auto/SYNC PRODUCER/CAN NODE/Bootup Frame generator/11-bit Adder/8-bit Adder/Half Adder ==
  A : Inport
  B : Inport  Port=2
  AND : Logic  IconShape=distinctive  AllPortsSameDT=off  OutDataTypeStr=boolean
  XOR1 : Logic  Operator=XOR  IconShape=distinctive  AllPortsSameDT=off  OutDataTypeStr=boolean
  S : Outport
  C : Outport  Port=2
  wires:
  A/1 -> XOR1/1, AND/1
  B/1 -> XOR1/2, AND/2
  AND/1 -> C/1
  XOR1/1 -> S/1

== system can8auto/SYNC PRODUCER/CAN NODE/NMT Frame generator/11-bit Adder/11-bit Adder/Full Adder ==
  A : Inport
  B : Inport  Port=2
  Cin : Inport  Port=3
  AND : Logic  IconShape=distinctive  AllPortsSameDT=off  OutDataTypeStr=boolean
  AND1 : Logic  IconShape=distinctive  AllPortsSameDT=off  OutDataTypeStr=boolean
  OR : Logic  Operator=OR  IconShape=distinctive  AllPortsSameDT=off  OutDataTypeStr=boolean
  XOR1 : Logic  Operator=XOR  IconShape=distinctive  AllPortsSameDT=off  OutDataTypeStr=boolean
  XOR2 : Logic  Operator=XOR  IconShape=distinctive  AllPortsSameDT=off  OutDataTypeStr=boolean
  S : Outport
  Cout : Outport  Port=2
  wires:
  AND/1 -> OR/1
  XOR2/1 -> S/1
  B/1 -> XOR1/2, AND1/2
  A/1 -> XOR1/1, AND1/1
  AND1/1 -> OR/2
  XOR1/1 -> XOR2/1, AND/2
  Cin/1 -> AND/1, XOR2/2
  OR/1 -> Cout/1

== system can8auto/SYNC PRODUCER/CAN NODE/NMT Frame generator/11-bit Adder/11-bit Adder/Full Adder1 ==
  A : Inport
  B : Inport  Port=2
  Cin : Inport  Port=3
  AND : Logic  IconShape=distinctive  AllPortsSameDT=off  OutDataTypeStr=boolean
  AND1 : Logic  IconShape=distinctive  AllPortsSameDT=off  OutDataTypeStr=boolean
  OR : Logic  Operator=OR  IconShape=distinctive  AllPortsSameDT=off  OutDataTypeStr=boolean
  XOR1 : Logic  Operator=XOR  IconShape=distinctive  AllPortsSameDT=off  OutDataTypeStr=boolean
  XOR2 : Logic  Operator=XOR  IconShape=distinctive  AllPortsSameDT=off  OutDataTypeStr=boolean
  S : Outport
  Cout : Outport  Port=2
  wires:
  AND/1 -> OR/1
  XOR2/1 -> S/1
  B/1 -> XOR1/2, AND1/2
  A/1 -> XOR1/1, AND1/1
  AND1/1 -> OR/2
  XOR1/1 -> XOR2/1, AND/2
  Cin/1 -> AND/1, XOR2/2
  OR/1 -> Cout/1

== system can8auto/SYNC PRODUCER/CAN NODE/NMT Frame generator/11-bit Adder/11-bit Adder/Full Adder2 ==
  A : Inport
  B : Inport  Port=2
  Cin : Inport  Port=3
  AND : Logic  IconShape=distinctive  AllPortsSameDT=off  OutDataTypeStr=boolean
  AND1 : Logic  IconShape=distinctive  AllPortsSameDT=off  OutDataTypeStr=boolean
  OR : Logic  Operator=OR  IconShape=distinctive  AllPortsSameDT=off  OutDataTypeStr=boolean
  XOR1 : Logic  Operator=XOR  IconShape=distinctive  AllPortsSameDT=off  OutDataTypeStr=boolean
  XOR2 : Logic  Operator=XOR  IconShape=distinctive  AllPortsSameDT=off  OutDataTypeStr=boolean
  S : Outport
  Cout : Outport  Port=2
  wires:
  AND/1 -> OR/1
  XOR2/1 -> S/1
  B/1 -> XOR1/2, AND1/2
  A/1 -> XOR1/1, AND1/1
  AND1/1 -> OR/2
  XOR1/1 -> XOR2/1, AND/2
  Cin/1 -> AND/1, XOR2/2
  OR/1 -> Cout/1

== system can8auto/SYNC PRODUCER/CAN NODE/NMT Frame generator/11-bit Adder/11-bit Adder/Full Adder3 ==
  A : Inport
  B : Inport  Port=2
  Cin : Inport  Port=3
  AND : Logic  IconShape=distinctive  AllPortsSameDT=off  OutDataTypeStr=boolean
  AND1 : Logic  IconShape=distinctive  AllPortsSameDT=off  OutDataTypeStr=boolean
  OR : Logic  Operator=OR  IconShape=distinctive  AllPortsSameDT=off  OutDataTypeStr=boolean
  XOR1 : Logic  Operator=XOR  IconShape=distinctive  AllPortsSameDT=off  OutDataTypeStr=boolean
  XOR2 : Logic  Operator=XOR  IconShape=distinctive  AllPortsSameDT=off  OutDataTypeStr=boolean
  S : Outport
  Cout : Outport  Port=2
  wires:
  AND/1 -> OR/1
  XOR2/1 -> S/1
  B/1 -> XOR1/2, AND1/2
  A/1 -> XOR1/1, AND1/1
  AND1/1 -> OR/2
  XOR1/1 -> XOR2/1, AND/2
  Cin/1 -> AND/1, XOR2/2
  OR/1 -> Cout/1

== system can8auto/SYNC PRODUCER/CAN NODE/NMT Frame generator/11-bit Adder/11-bit Adder/Full Adder4 ==
  A : Inport
  B : Inport  Port=2
  Cin : Inport  Port=3
  AND : Logic  IconShape=distinctive  AllPortsSameDT=off  OutDataTypeStr=boolean
  AND1 : Logic  IconShape=distinctive  AllPortsSameDT=off  OutDataTypeStr=boolean
  OR : Logic  Operator=OR  IconShape=distinctive  AllPortsSameDT=off  OutDataTypeStr=boolean
  XOR1 : Logic  Operator=XOR  IconShape=distinctive  AllPortsSameDT=off  OutDataTypeStr=boolean
  XOR2 : Logic  Operator=XOR  IconShape=distinctive  AllPortsSameDT=off  OutDataTypeStr=boolean
  S : Outport
  Cout : Outport  Port=2
  wires:
  AND/1 -> OR/1
  XOR2/1 -> S/1
  B/1 -> XOR1/2, AND1/2
  A/1 -> XOR1/1, AND1/1
  AND1/1 -> OR/2
  XOR1/1 -> XOR2/1, AND/2
  Cin/1 -> AND/1, XOR2/2
  OR/1 -> Cout/1

== system can8auto/SYNC PRODUCER/CAN NODE/NMT Frame generator/11-bit Adder/11-bit Adder/Full Adder5 ==
  A : Inport
  B : Inport  Port=2
  Cin : Inport  Port=3
  AND : Logic  IconShape=distinctive  AllPortsSameDT=off  OutDataTypeStr=boolean
  AND1 : Logic  IconShape=distinctive  AllPortsSameDT=off  OutDataTypeStr=boolean
  OR : Logic  Operator=OR  IconShape=distinctive  AllPortsSameDT=off  OutDataTypeStr=boolean
  XOR1 : Logic  Operator=XOR  IconShape=distinctive  AllPortsSameDT=off  OutDataTypeStr=boolean
  XOR2 : Logic  Operator=XOR  IconShape=distinctive  AllPortsSameDT=off  OutDataTypeStr=boolean
  S : Outport
  Cout : Outport  Port=2
  wires:
  AND/1 -> OR/1
  XOR2/1 -> S/1
  B/1 -> XOR1/2, AND1/2
  A/1 -> XOR1/1, AND1/1
  AND1/1 -> OR/2
  XOR1/1 -> XOR2/1, AND/2
  Cin/1 -> AND/1, XOR2/2
  OR/1 -> Cout/1

== system can8auto/SYNC PRODUCER/CAN NODE/NMT Frame generator/11-bit Adder/11-bit Adder/Full Adder6 ==
  A : Inport
  B : Inport  Port=2
  Cin : Inport  Port=3
  AND : Logic  IconShape=distinctive  AllPortsSameDT=off  OutDataTypeStr=boolean
  AND1 : Logic  IconShape=distinctive  AllPortsSameDT=off  OutDataTypeStr=boolean
  OR : Logic  Operator=OR  IconShape=distinctive  AllPortsSameDT=off  OutDataTypeStr=boolean
  XOR1 : Logic  Operator=XOR  IconShape=distinctive  AllPortsSameDT=off  OutDataTypeStr=boolean
  XOR2 : Logic  Operator=XOR  IconShape=distinctive  AllPortsSameDT=off  OutDataTypeStr=boolean
  S : Outport
  Cout : Outport  Port=2
  wires:
  AND/1 -> OR/1
  XOR2/1 -> S/1
  B/1 -> XOR1/2, AND1/2
  A/1 -> XOR1/1, AND1/1
  AND1/1 -> OR/2
  XOR1/1 -> XOR2/1, AND/2
  Cin/1 -> AND/1, XOR2/2
  OR/1 -> Cout/1

== system can8auto/SYNC PRODUCER/CAN NODE/NMT Frame generator/11-bit Adder/11-bit Adder/Full Adder7 ==
  A : Inport
  B : Inport  Port=2
  Cin : Inport  Port=3
  AND : Logic  IconShape=distinctive  AllPortsSameDT=off  OutDataTypeStr=boolean
  AND1 : Logic  IconShape=distinctive  AllPortsSameDT=off  OutDataTypeStr=boolean
  OR : Logic  Operator=OR  IconShape=distinctive  AllPortsSameDT=off  OutDataTypeStr=boolean
  XOR1 : Logic  Operator=XOR  IconShape=distinctive  AllPortsSameDT=off  OutDataTypeStr=boolean
  XOR2 : Logic  Operator=XOR  IconShape=distinctive  AllPortsSameDT=off  OutDataTypeStr=boolean
  S : Outport
  Cout : Outport  Port=2
  wires:
  AND/1 -> OR/1
  XOR2/1 -> S/1
  B/1 -> XOR1/2, AND1/2
  A/1 -> XOR1/1, AND1/1
  AND1/1 -> OR/2
  XOR1/1 -> XOR2/1, AND/2
  Cin/1 -> AND/1, XOR2/2
  OR/1 -> Cout/1

== system can8auto/SYNC PRODUCER/CAN NODE/NMT Frame generator/11-bit Adder/11-bit Adder/Full Adder8 ==
  A : Inport
  B : Inport  Port=2
  Cin : Inport  Port=3
  AND : Logic  IconShape=distinctive  AllPortsSameDT=off  OutDataTypeStr=boolean
  AND1 : Logic  IconShape=distinctive  AllPortsSameDT=off  OutDataTypeStr=boolean
  OR : Logic  Operator=OR  IconShape=distinctive  AllPortsSameDT=off  OutDataTypeStr=boolean
  XOR1 : Logic  Operator=XOR  IconShape=distinctive  AllPortsSameDT=off  OutDataTypeStr=boolean
  XOR2 : Logic  Operator=XOR  IconShape=distinctive  AllPortsSameDT=off  OutDataTypeStr=boolean
  S : Outport
  Cout : Outport  Port=2
  wires:
  AND/1 -> OR/1
  XOR2/1 -> S/1
  B/1 -> XOR1/2, AND1/2
  A/1 -> XOR1/1, AND1/1
  AND1/1 -> OR/2
  XOR1/1 -> XOR2/1, AND/2
  Cin/1 -> AND/1, XOR2/2
  OR/1 -> Cout/1

== system can8auto/SYNC PRODUCER/CAN NODE/NMT Frame generator/11-bit Adder/11-bit Adder/Full Adder9 ==
  A : Inport
  B : Inport  Port=2
  Cin : Inport  Port=3
  AND : Logic  IconShape=distinctive  AllPortsSameDT=off  OutDataTypeStr=boolean
  AND1 : Logic  IconShape=distinctive  AllPortsSameDT=off  OutDataTypeStr=boolean
  OR : Logic  Operator=OR  IconShape=distinctive  AllPortsSameDT=off  OutDataTypeStr=boolean
  XOR1 : Logic  Operator=XOR  IconShape=distinctive  AllPortsSameDT=off  OutDataTypeStr=boolean
  XOR2 : Logic  Operator=XOR  IconShape=distinctive  AllPortsSameDT=off  OutDataTypeStr=boolean
  S : Outport
  Cout : Outport  Port=2
  wires:
  AND/1 -> OR/1
  XOR2/1 -> S/1
  B/1 -> XOR1/2, AND1/2
  A/1 -> XOR1/1, AND1/1
  AND1/1 -> OR/2
  XOR1/1 -> XOR2/1, AND/2
  Cin/1 -> AND/1, XOR2/2
  OR/1 -> Cout/1

== system can8auto/SYNC PRODUCER/CAN NODE/NMT Frame generator/11-bit Adder/11-bit Adder/Half Adder ==
  A : Inport
  B : Inport  Port=2
  AND : Logic  IconShape=distinctive  AllPortsSameDT=off  OutDataTypeStr=boolean
  XOR1 : Logic  Operator=XOR  IconShape=distinctive  AllPortsSameDT=off  OutDataTypeStr=boolean
  S : Outport
  C : Outport  Port=2
  wires:
  A/1 -> XOR1/1, AND/1
  B/1 -> XOR1/2, AND/2
  AND/1 -> C/1
  XOR1/1 -> S/1

== matlab function can8auto/CAN MASTER/CAN NODE/Bootup Frame generator/BitStuffing/MATLAB Function ==
  data: u input; b output
function b = fcn(u)
a = u;
b = zeros(1,floor(length(a)+length(a)/5));
k = 0;
count2 = 1;
i = 1;
n = length(a);
count = 1;
j = 1;
while i < n
    if a(i) == 1
        b(j) = a(i);
        while a(i+1) == 1 && i+1 < n && count < 5
            j = j+1;
            b(j) = a(i+1);
            count = count + 1;
            count2 = count;
            if count == 5
                j = j+1;
                b(j) = 0;
            end
            i = i+1;
        end
        
    else
        b(j) = a(i);
    end
    
    if a(i) == 0
    if a(i) == 0
        b(j) = a(i);
        while a(i+1) == 0 && i+1 < n && count < 5
            j = j+1;
            b(j) = a(i+1);
            count = count + 1;
            count2 = count;
            if count == 5
                j = j+1;
                b(j) = 1;
            end
            i = i+1;
        end
        
    else
        b(j) = a(i);
    end
    end
    
    i = i+1;
    j = j+1;
    count = 1;
end
if i == n && a(i) == 1 && count2 == 4
    b(j) = a(i);
    b(j+1) = 0;
else
    b(j) = a(i);
end

if i == n && a(i) == 0 && count2 == 4
    b(j) = a(i);
    b(j+1) = 1;
else
    b(j) = a(i);
end

== matlab function can8auto/PDO NODO CAN /MATLAB Function2 ==
  data: u input; y output
function y = fcn(u)
    if u > 0
        y = 1;
    else
        y = 0;
    end
end

== matlab function can8auto/CAN MASTER/CAN NODE/Frame MUX/MATLAB Function2 ==
  data: mode input; result output size=[1 200]; u1 input; size input
function result = MUX_lv2(mode, u1, size)
%#codegen
%
% Insert zeros between elements

switch mode
    case 0
        result = u1(1 : size(1));
    case 1
        result = u1(size(1)+1 : size(1)+size(2));
    case 2
        result = u1(size(1)+size(2)+1 : size(1)+size(2)+size(3));
    case 3
        result = u1(size(1)+size(2)+size(3)+1 : size(1)+size(2)+size(3)+size(4));
    otherwise
        result = u1(size(1)+size(2)+size(3)+size(4)+1 : size(1)+size(2)+size(3)+size(4)+size(5));
end

== matlab function can8auto/CAN MASTER/CAN NODE/NMT Frame generator/BitStuffing/MATLAB Function ==
  data: u input; b output
function b = fcn(u)
a = u;
b = zeros(1,floor(length(a)+length(a)/5));
k = 0;
count2 = 1;
i = 1;
n = length(a);
count = 1;
j = 1;
while i < n
    if a(i) == 1
        b(j) = a(i);
        while a(i+1) == 1 && i+1 < n && count < 5
            j = j+1;
            b(j) = a(i+1);
            count = count + 1;
            count2 = count;
            if count == 5
                j = j+1;
                b(j) = 0;
            end
            i = i+1;
        end
        
    else
        b(j) = a(i);
    end
    
    if a(i) == 0
    if a(i) == 0
        b(j) = a(i);
        while a(i+1) == 0 && i+1 < n && count < 5
            j = j+1;
            b(j) = a(i+1);
            count = count + 1;
            count2 = count;
            if count == 5
                j = j+1;
                b(j) = 1;
            end
            i = i+1;
        end
        
    else
        b(j) = a(i);
    end
    end
    
    i = i+1;
    j = j+1;
    count = 1;
end
if i == n && a(i) == 1 && count2 == 4
    b(j) = a(i);
    b(j+1) = 0;
else
    b(j) = a(i);
end

if i == n && a(i) == 0 && count2 == 4
    b(j) = a(i);
    b(j+1) = 1;
else
    b(j) = a(i);
end

== matlab function can8auto/SDO NODO CAN/CAN NODE/Bootup Frame generator/BitStuffing/MATLAB Function ==
  data: u input; b output
function b = fcn(u)
a = u;
b = zeros(1,floor(length(a)+length(a)/5));
k = 0;
count2 = 1;
i = 1;
n = length(a);
count = 1;
j = 1;
while i < n
    if a(i) == 1
        b(j) = a(i);
        while a(i+1) == 1 && i+1 < n && count < 5
            j = j+1;
            b(j) = a(i+1);
            count = count + 1;
            count2 = count;
            if count == 5
                j = j+1;
                b(j) = 0;
            end
            i = i+1;
        end
        
    else
        b(j) = a(i);
    end
    
    if a(i) == 0
    if a(i) == 0
        b(j) = a(i);
        while a(i+1) == 0 && i+1 < n && count < 5
            j = j+1;
            b(j) = a(i+1);
            count = count + 1;
            count2 = count;
            if count == 5
                j = j+1;
                b(j) = 1;
            end
            i = i+1;
        end
        
    else
        b(j) = a(i);
    end
    end
    
    i = i+1;
    j = j+1;
    count = 1;
end
if i == n && a(i) == 1 && count2 == 4
    b(j) = a(i);
    b(j+1) = 0;
else
    b(j) = a(i);
end

if i == n && a(i) == 0 && count2 == 4
    b(j) = a(i);
    b(j+1) = 1;
else
    b(j) = a(i);
end

== matlab function can8auto/SDO NODO CAN/CAN NODE/Frame MUX/MATLAB Function2 ==
  data: mode input; result output size=[1 200]; u1 input; size input
function result = MUX_lv2(mode, u1, size)
%#codegen
%
% Insert zeros between elements

switch mode
    case 0
        result = u1(1 : size(1));
    case 1
        result = u1(size(1)+1 : size(1)+size(2));
    case 2
        result = u1(size(1)+size(2)+1 : size(1)+size(2)+size(3));
    case 3
        result = u1(size(1)+size(2)+size(3)+1 : size(1)+size(2)+size(3)+size(4));
    otherwise
        result = u1(size(1)+size(2)+size(3)+size(4)+1 : size(1)+size(2)+size(3)+size(4)+size(5));
end

== matlab function can8auto/SDO NODO CAN/CAN NODE/NMT Frame generator/BitStuffing/MATLAB Function ==
  data: u input; b output
function b = fcn(u)
a = u;
b = zeros(1,floor(length(a)+length(a)/5));
k = 0;
count2 = 1;
i = 1;
n = length(a);
count = 1;
j = 1;
while i < n
    if a(i) == 1
        b(j) = a(i);
        while a(i+1) == 1 && i+1 < n && count < 5
            j = j+1;
            b(j) = a(i+1);
            count = count + 1;
            count2 = count;
            if count == 5
                j = j+1;
                b(j) = 0;
            end
            i = i+1;
        end
        
    else
        b(j) = a(i);
    end
    
    if a(i) == 0
    if a(i) == 0
        b(j) = a(i);
        while a(i+1) == 0 && i+1 < n && count < 5
            j = j+1;
            b(j) = a(i+1);
            count = count + 1;
            count2 = count;
            if count == 5
                j = j+1;
                b(j) = 1;
            end
            i = i+1;
        end
        
    else
        b(j) = a(i);
    end
    end
    
    i = i+1;
    j = j+1;
    count = 1;
end
if i == n && a(i) == 1 && count2 == 4
    b(j) = a(i);
    b(j+1) = 0;
else
    b(j) = a(i);
end

if i == n && a(i) == 0 && count2 == 4
    b(j) = a(i);
    b(j+1) = 1;
else
    b(j) = a(i);
end

== matlab function can8auto/CAN MASTER/CAN NODE/SDO Frame generator/BitStuffing/MATLAB Function ==
  data: u input; b output
function b = fcn(u)
a = u;
b = zeros(1,floor(length(a)+length(a)/5));
k = 0;
count2 = 1;
i = 1;
n = length(a);
count = 1;
j = 1;
while i < n
    if a(i) == 1
        b(j) = a(i);
        while a(i+1) == 1 && i+1 < n && count < 5
            j = j+1;
            b(j) = a(i+1);
            count = count + 1;
            count2 = count;
            if count == 5
                j = j+1;
                b(j) = 0;
            end
            i = i+1;
        end
        
    else
        b(j) = a(i);
    end
    
    if a(i) == 0
    if a(i) == 0
        b(j) = a(i);
        while a(i+1) == 0 && i+1 < n && count < 5
            j = j+1;
            b(j) = a(i+1);
            count = count + 1;
            count2 = count;
            if count == 5
                j = j+1;
                b(j) = 1;
            end
            i = i+1;
        end
        
    else
        b(j) = a(i);
    end
    end
    
    i = i+1;
    j = j+1;
    count = 1;
end
if i == n && a(i) == 1 && count2 == 4
    b(j) = a(i);
    b(j+1) = 0;
else
    b(j) = a(i);
end

if i == n && a(i) == 0 && count2 == 4
    b(j) = a(i);
    b(j+1) = 1;
else
    b(j) = a(i);
end

== matlab function can8auto/CAN MASTER/CAN NODE/SDO Frame generator/MUX/MATLAB Function ==
  data: index input; result output size=[1 64]; u1 input
function result  = mux(index, u1)
%#codegen
%
% Insert zeros between elements

result = zeros(1,64);
switch index
    case 0
        result = u1(1:64);
    case 1
        result = u1(65:128);
    case 2
        result = u1(129:192);
    otherwise
        result = u1(193:256);
end

== matlab function can8auto/CAN MASTER/CAN NODE/SYNC Frame Generator/BitStuffing/MATLAB Function ==
  data: u input; b output
function b = fcn(u)
a = u;
b = zeros(1,floor(length(a)+length(a)/5));
k = 0;
count2 = 1;
i = 1;
n = length(a);
count = 1;
j = 1;
while i < n
    if a(i) == 1
        b(j) = a(i);
        while a(i+1) == 1 && i+1 < n && count < 5
            j = j+1;
            b(j) = a(i+1);
            count = count + 1;
            count2 = count;
            if count == 5
                j = j+1;
                b(j) = 0;
            end
            i = i+1;
        end
        
    else
        b(j) = a(i);
    end
    
    if a(i) == 0
    if a(i) == 0
        b(j) = a(i);
        while a(i+1) == 0 && i+1 < n && count < 5
            j = j+1;
            b(j) = a(i+1);
            count = count + 1;
            count2 = count;
            if count == 5
                j = j+1;
                b(j) = 1;
            end
            i = i+1;
        end
        
    else
        b(j) = a(i);
    end
    end
    
    i = i+1;
    j = j+1;
    count = 1;
end
if i == n && a(i) == 1 && count2 == 4
    b(j) = a(i);
    b(j+1) = 0;
else
    b(j) = a(i);
end

if i == n && a(i) == 0 && count2 == 4
    b(j) = a(i);
    b(j+1) = 1;
else
    b(j) = a(i);
end

== stateflow chart can8auto/CAN MASTER/Chart ==
  state NoTX
    entry: state = 0;
  state SenseBus
    entry: state = 1;
  state TXcompleated
    entry: state = 4;
  state TX
    entry: state = 2;
  NoTX -> NoTX [order 2] : [Frame == 0]
  (default) -> NoTX
  SenseBus -> SenseBus [order 1] : [Free == 0 || EndTX == 1]
  TXcompleated -> NoTX [order 1] : [Frame == 0]
  NoTX -> SenseBus [order 1] : [Frame  > 0]
  TX -> SenseBus [order 2] : [Error == 1]
  TXcompleated -> SenseBus [order 2] : [Frame  > 0]
  SenseBus -> TX [order 2] : [Free == 1]
  TX -> TXcompleated [order 1] : [EndTX == 1]
  TX -> TX [order 3]
  data: Free input; Error input; Frame input; EndTX input; state output
